simulink library "AeroSim"  (Simulink 7.8)
settings: Solver=ode45  StartTime=0.0  StopTime=10.0  RelTol=1e-3
libraries: AeroSim x13
settings Model: Creator=Ryan  LastModifiedBy=Ryan

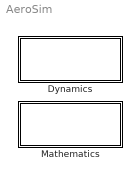
== system AeroSim ==
  Dynamics : Subsystem
      mask Display: disp('Dynamics')
  Mathematics : Subsystem
      mask Display: disp('Mathematics')

== system AeroSim/Dynamics ==
  Equations of Motion : Subsystem
  Rotational EoM : Subsystem
  Translational EoM : Subsystem

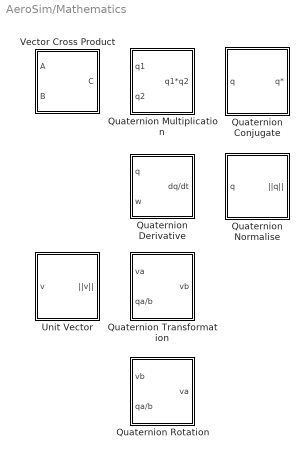
== system AeroSim/Mathematics ==
  Quaternion Conjugate : Subsystem
  Quaternion Derivative : Subsystem
  Quaternion Multiplication : Subsystem
  Quaternion Normalise : Subsystem
  Quaternion Rotation : Subsystem
  Quaternion Transformation : Subsystem
  Unit Vector : Subsystem
  Vector Cross Product : Subsystem

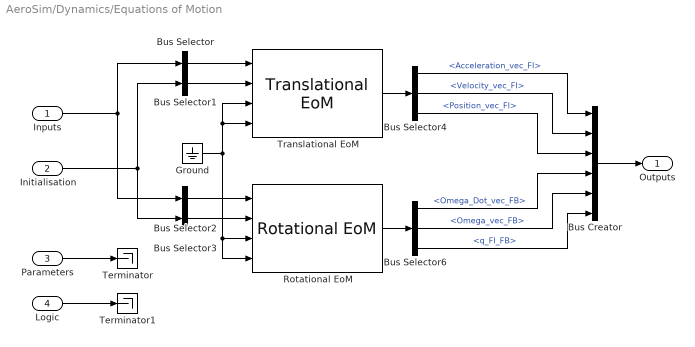
== system AeroSim/Dynamics/Equations of Motion ==
  Inputs : Inport  OutDataTypeStr=Bus: Dynamics_EquationsOfMotion_Inputs
  Initialisation : Inport  Port=2  OutDataTypeStr=Bus: Dynamics_EquationsOfMotion_Initialisation
  Parameters : Inport  Port=3
  Logic : Inport  Port=4
  Bus Creator : BusCreator  Inputs=6
  Bus Selector : BusSelector  OutputSignals=Force_vec_FI,Mass  OutputAsBus=on
  Bus Selector1 : BusSelector  OutputSignals=Ini_Velocity_vec_FI,Ini_Position_vec_FI  OutputAsBus=on
  Bus Selector2 : BusSelector  OutputSignals=Torque_vec_FB,Inertia_mat_FB  OutputAsBus=on
  Bus Selector3 : BusSelector  OutputSignals=Ini_Omega_vec_FB,Ini_q_FI_FB  OutputAsBus=on
  Bus Selector4 : BusSelector  OutputSignals=Acceleration_vec_FI,Velocity_vec_FI,Position_vec_FI
  Bus Selector6 : BusSelector  OutputSignals=Omega_Dot_vec_FB,Omega_vec_FB,q_FI_FB
  Ground : Ground
  Rotational EoM : AeroSim/Dynamics/Rotational EoM
  Terminator : Terminator
  Terminator1 : Terminator
  Translational EoM : AeroSim/Dynamics/Translational EoM
  Outputs : Outport  OutDataTypeStr=Bus: Dynamics_EquationsOfMotion_Outputs
  wires:
  Ground/1 -> Rotational EoM/4, Rotational EoM/3, Translational EoM/4, Translational EoM/3
  Bus Selector3/1 -> Rotational EoM/2
  Bus Selector2/1 -> Rotational EoM/1
  Initialisation/1 -> Bus Selector3/1, Bus Selector1/1
  Bus Selector1/1 -> Translational EoM/2
  Bus Selector/1 -> Translational EoM/1
  Inputs/1 -> Bus Selector2/1, Bus Selector/1
  Bus Creator/1 -> Outputs/1
  Bus Selector4/3 -> Bus Creator/3  "<Position_vec_FI>"
  Bus Selector4/2 -> Bus Creator/2  "<Velocity_vec_FI>"
  Bus Selector4/1 -> Bus Creator/1  "<Acceleration_vec_FI>"
  Bus Selector6/3 -> Bus Creator/6  "<q_FI_FB>"
  Bus Selector6/2 -> Bus Creator/5  "<Omega_vec_FB>"
  Bus Selector6/1 -> Bus Creator/4  "<Omega_Dot_vec_FB>"
  Rotational EoM/1 -> Bus Selector6/1
  Translational EoM/1 -> Bus Selector4/1
  Logic/1 -> Terminator1/1
  Parameters/1 -> Terminator/1

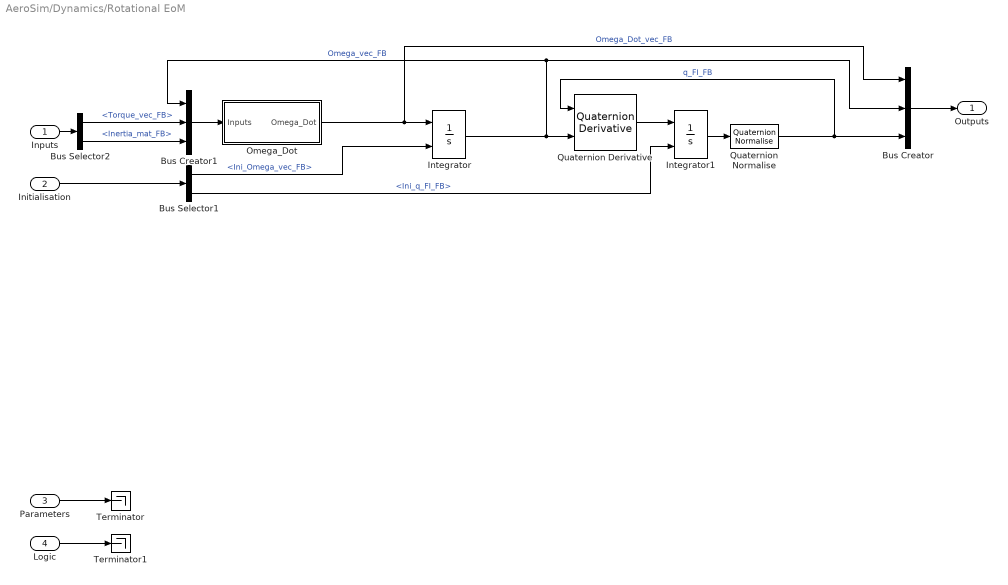
== system AeroSim/Dynamics/Rotational EoM ==
  Inputs : Inport  OutDataTypeStr=Bus: Dynamics_RotationalEoM_Inputs
  Initialisation : Inport  Port=2  OutDataTypeStr=Bus: Dynamics_RotationalEoM_Initialisation
  Parameters : Inport  Port=3
  Logic : Inport  Port=4
  Bus Creator : BusCreator  Inputs=3
  Bus Creator1 : BusCreator  Inputs=3
  Bus Selector1 : BusSelector  OutputSignals=Ini_Omega_vec_FB,Ini_q_FI_FB
  Bus Selector2 : BusSelector  OutputSignals=Torque_vec_FB,Inertia_mat_FB
  Integrator : Integrator  InitialConditionSource=external
  Integrator1 : Integrator  InitialConditionSource=external
  Omega_Dot : Subsystem
  Quaternion Derivative : AeroSim/Mathematics/Quaternion Derivative
  Quaternion Normalise : AeroSim/Mathematics/Quaternion Normalise
  Terminator : Terminator
  Terminator1 : Terminator
  Outputs : Outport  OutDataTypeStr=Bus: Dynamics_RotationalEoM_Outputs
  wires:
  Bus Creator1/1 -> Omega_Dot/1(Inputs)
  Bus Selector2/1 -> Bus Creator1/2  "<Torque_vec_FB>"
  Bus Selector2/2 -> Bus Creator1/3  "<Inertia_mat_FB>"
  Inputs/1 -> Bus Selector2/1
  Quaternion Normalise/1 -> Bus Creator/3, Quaternion Derivative/1  "q_FI_FB"
  Integrator1/1 -> Quaternion Normalise/1
  Bus Selector1/2 -> Integrator1/2  "<Ini_q_FI_FB>"
  Quaternion Derivative/1 -> Integrator1/1
  Integrator/1 -> Bus Creator1/1, Bus Creator/2, Quaternion Derivative/2  "Omega_vec_FB"
  Bus Selector1/1 -> Integrator/2  "<Ini_Omega_vec_FB>"
  Omega_Dot/1(Omega_Dot) -> Bus Creator/1, Integrator/1  "Omega_Dot_vec_FB"
  Bus Creator/1 -> Outputs/1
  Initialisation/1 -> Bus Selector1/1
  Logic/1 -> Terminator1/1
  Parameters/1 -> Terminator/1

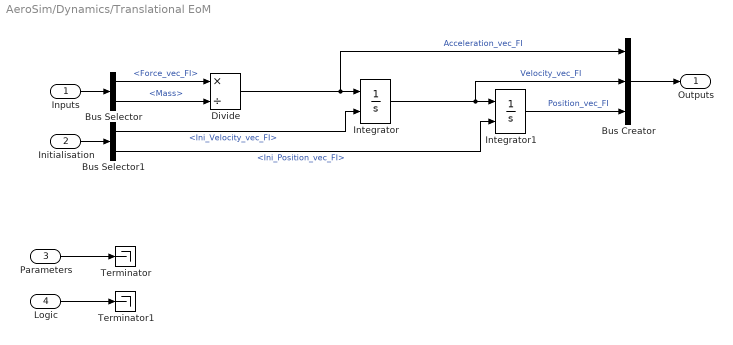
== system AeroSim/Dynamics/Translational EoM ==
  Inputs : Inport  OutDataTypeStr=Bus: Dynamics_TranslationalEoM_Inputs
  Initialisation : Inport  Port=2  OutDataTypeStr=Bus: Dynamics_TranslationalEoM_Initialisation
  Parameters : Inport  Port=3
  Logic : Inport  Port=4
  Bus Creator : BusCreator  Inputs=3
  Bus Selector : BusSelector  OutputSignals=Force_vec_FI,Mass
  Bus Selector1 : BusSelector  OutputSignals=Ini_Velocity_vec_FI,Ini_Position_vec_FI
  Divide : Product  Inputs=*/
  Integrator : Integrator  InitialConditionSource=external
  Integrator1 : Integrator  InitialConditionSource=external
  Terminator : Terminator
  Terminator1 : Terminator
  Outputs : Outport  OutDataTypeStr=Bus: Dynamics_TranslationalEoM_Outputs
  wires:
  Parameters/1 -> Terminator/1
  Logic/1 -> Terminator1/1
  Inputs/1 -> Bus Selector/1
  Bus Selector/1 -> Divide/1  "<Force_vec_FI>"
  Bus Selector/2 -> Divide/2  "<Mass>"
  Initialisation/1 -> Bus Selector1/1
  Bus Creator/1 -> Outputs/1
  Divide/1 -> Integrator/1, Bus Creator/1  "Acceleration_vec_FI"
  Bus Selector1/1 -> Integrator/2  "<Ini_Velocity_vec_FI>"
  Integrator/1 -> Integrator1/1, Bus Creator/2  "Velocity_vec_FI"
  Bus Selector1/2 -> Integrator1/2  "<Ini_Position_vec_FI>"
  Integrator1/1 -> Bus Creator/3  "Position_vec_FI"

== system AeroSim/Mathematics/Quaternion Conjugate ==
  q : Inport
  Demux : Demux  Outputs=[1 3]
  Gain : Gain  Gain=-1
  Mux : Mux  Inputs=2
  q* : Outport
  wires:
  q/1 -> Demux/1
  Demux/2 -> Gain/1
  Demux/1 -> Mux/1
  Gain/1 -> Mux/2
  Mux/1 -> q*/1

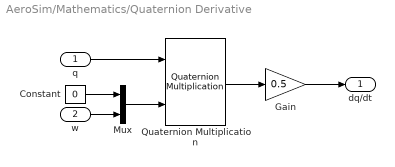
== system AeroSim/Mathematics/Quaternion Derivative ==
  q : Inport
  w : Inport  Port=2
  Constant : Constant  Value=0
  Gain : Gain  Gain=0.5
  Mux : Mux  Inputs=2
  Quaternion Multiplication : AeroSim/Mathematics/Quaternion Multiplication
  dq/dt : Outport
  wires:
  w/1 -> Mux/2
  Constant/1 -> Mux/1
  q/1 -> Quaternion Multiplication/1
  Mux/1 -> Quaternion Multiplication/2
  Quaternion Multiplication/1 -> Gain/1
  Gain/1 -> dq/dt/1

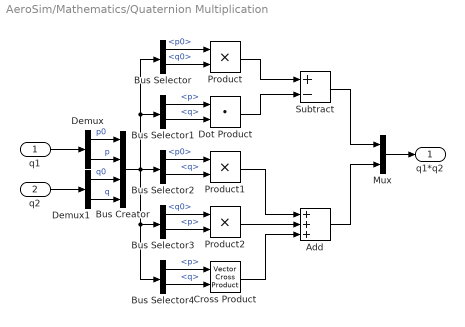
== system AeroSim/Mathematics/Quaternion Multiplication ==
  q1 : Inport
  q2 : Inport  Port=2
  Add : Sum  Inputs=+++
  Bus Creator : BusCreator
  Bus Selector : BusSelector  OutputSignals=p0,q0
  Bus Selector1 : BusSelector  OutputSignals=p,q
  Bus Selector2 : BusSelector  OutputSignals=p0,q
  Bus Selector3 : BusSelector  OutputSignals=q0,p
  Bus Selector4 : BusSelector  OutputSignals=p,q
  Cross Product : AeroSim/Mathematics/Vector Cross Product
  Demux : Demux  Outputs=[1 3]
  Demux1 : Demux  Outputs=[1 3]
  Dot Product : DotProduct  InputSameDT=on  OutDataTypeStr=Inherit: Inherit via internal rule
  Mux : Mux  Inputs=2
  Product : Product  RndMeth=Zero
  Product1 : Product  RndMeth=Zero
  Product2 : Product  RndMeth=Zero
  Subtract : Sum  Inputs=+-
  q1*q2 : Outport
  wires:
  q1/1 -> Demux/1
  q2/1 -> Demux1/1
  Product/1 -> Subtract/1
  Dot Product/1 -> Subtract/2
  Product2/1 -> Add/2
  Product1/1 -> Add/1
  Cross Product/1 -> Add/3
  Subtract/1 -> Mux/1
  Add/1 -> Mux/2
  Mux/1 -> q1*q2/1
  Demux/1 -> Bus Creator/1  "p0"
  Demux/2 -> Bus Creator/2  "p"
  Demux1/1 -> Bus Creator/3  "q0"
  Demux1/2 -> Bus Creator/4  "q"
  Bus Selector/1 -> Product/1  "<p0>"
  Bus Selector/2 -> Product/2  "<q0>"
  Bus Creator/1 -> Bus Selector2/1, Bus Selector/1, Bus Selector1/1, Bus Selector3/1, Bus Selector4/1
  Bus Selector1/1 -> Dot Product/1  "<p>"
  Bus Selector1/2 -> Dot Product/2  "<q>"
  Bus Selector2/1 -> Product1/1  "<p0>"
  Bus Selector2/2 -> Product1/2  "<q>"
  Bus Selector3/1 -> Product2/1  "<q0>"
  Bus Selector3/2 -> Product2/2  "<p>"
  Bus Selector4/1 -> Cross Product/1  "<p>"
  Bus Selector4/2 -> Cross Product/2  "<q>"

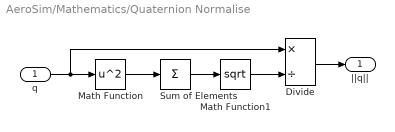
== system AeroSim/Mathematics/Quaternion Normalise ==
  q : Inport
  Divide : Product  Inputs=*/
  Math Function : Math  Operator=square  SaturateOnIntegerOverflow=on
  Math Function1 : Math  Operator=sqrt  SaturateOnIntegerOverflow=on
  Sum of Elements : Sum  Inputs=+
  ||q|| : Outport
  wires:
  q/1 -> Divide/1, Math Function/1
  Divide/1 -> ||q||/1
  Math Function1/1 -> Divide/2
  Sum of Elements/1 -> Math Function1/1
  Math Function/1 -> Sum of Elements/1

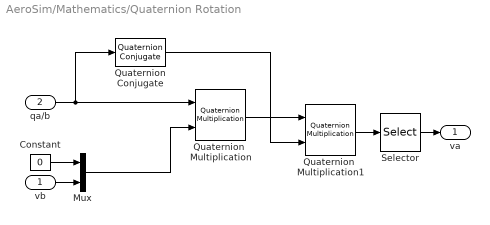
== system AeroSim/Mathematics/Quaternion Rotation ==
  vb : Inport
  qa/b : Inport  Port=2
  Constant : Constant  Value=0
  Mux : Mux  Inputs=2
  Quaternion Conjugate : AeroSim/Mathematics/Quaternion Conjugate
  Quaternion  Multiplication : AeroSim/Mathematics/Quaternion Multiplication
  Quaternion  Multiplication1 : AeroSim/Mathematics/Quaternion Multiplication
  Selector : Selector  InputPortWidth=4  IndexOptions=Index vector (dialog)  Indices=[2 3 4]  OutputSizes=1
  va : Outport
  wires:
  vb/1 -> Mux/2
  Constant/1 -> Mux/1
  qa/b/1 -> Quaternion  Multiplication/1, Quaternion Conjugate/1
  Mux/1 -> Quaternion  Multiplication/2
  Quaternion  Multiplication/1 -> Quaternion  Multiplication1/1
  Quaternion  Multiplication1/1 -> Selector/1
  Selector/1 -> va/1
  Quaternion Conjugate/1 -> Quaternion  Multiplication1/2

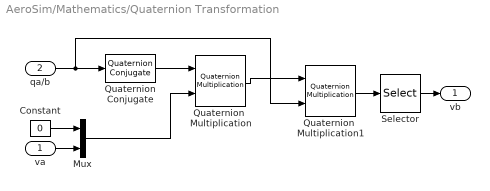
== system AeroSim/Mathematics/Quaternion Transformation ==
  va : Inport
  qa/b : Inport  Port=2
  Constant : Constant  Value=0
  Mux : Mux  Inputs=2
  Quaternion Conjugate : AeroSim/Mathematics/Quaternion Conjugate
  Quaternion  Multiplication : AeroSim/Mathematics/Quaternion Multiplication
  Quaternion  Multiplication1 : AeroSim/Mathematics/Quaternion Multiplication
  Selector : Selector  InputPortWidth=4  IndexOptions=Index vector (dialog)  Indices=[2 3 4]  OutputSizes=1
  vb : Outport
  wires:
  va/1 -> Mux/2
  Constant/1 -> Mux/1
  qa/b/1 -> Quaternion Conjugate/1, Quaternion  Multiplication1/2
  Mux/1 -> Quaternion  Multiplication/2
  Quaternion Conjugate/1 -> Quaternion  Multiplication/1
  Quaternion  Multiplication/1 -> Quaternion  Multiplication1/1
  Quaternion  Multiplication1/1 -> Selector/1
  Selector/1 -> vb/1

== system AeroSim/Mathematics/Unit Vector ==
  v : Inport
  Divide : Product  Inputs=*/
  Math Function : Math  Operator=square  SaturateOnIntegerOverflow=on
  Math Function1 : Math  Operator=sqrt  SaturateOnIntegerOverflow=on
  Sum of Elements : Sum  Inputs=+
  ||v|| : Outport
  wires:
  v/1 -> Divide/1, Math Function/1
  Divide/1 -> ||v||/1
  Math Function1/1 -> Divide/2
  Sum of Elements/1 -> Math Function1/1
  Math Function/1 -> Sum of Elements/1

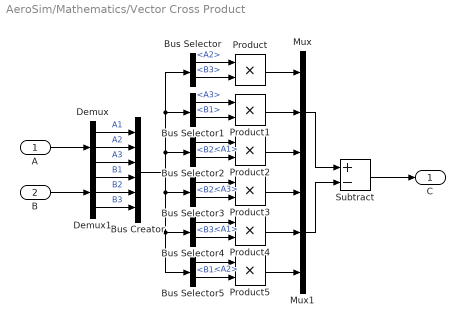
== system AeroSim/Mathematics/Vector Cross Product ==
  A : Inport
  B : Inport  Port=2
  Bus Creator : BusCreator  Inputs=6
  Bus Selector : BusSelector  OutputSignals=A2,B3
  Bus Selector1 : BusSelector  OutputSignals=A3,B1
  Bus Selector2 : BusSelector  OutputSignals=A1,B2
  Bus Selector3 : BusSelector  OutputSignals=A3,B2
  Bus Selector4 : BusSelector  OutputSignals=A1,B3
  Bus Selector5 : BusSelector  OutputSignals=A2,B1
  Demux : Demux  Outputs=3
  Demux1 : Demux  Outputs=3
  Mux : Mux  Inputs=3
  Mux1 : Mux  Inputs=3
  Product{,1..5} (6 alike) : Product  RndMeth=Zero
  Subtract : Sum  Inputs=+-
  C : Outport
  wires:
  Subtract/1 -> C/1
  Bus Creator/1 -> Bus Selector4/1, Bus Selector5/1, Bus Selector3/1, Bus Selector2/1, Bus Selector1/1, Bus Selector/1
  Mux1/1 -> Subtract/2
  Mux/1 -> Subtract/1
  Product5/1 -> Mux1/3
  Product4/1 -> Mux1/2
  Product3/1 -> Mux1/1
  Product2/1 -> Mux/3
  Product1/1 -> Mux/2
  Product/1 -> Mux/1
  Bus Selector5/2 -> Product5/2  "<B1>"
  Bus Selector5/1 -> Product5/1  "<A2>"
  Bus Selector4/2 -> Product4/2  "<B3>"
  Bus Selector4/1 -> Product4/1  "<A1>"
  Bus Selector3/2 -> Product3/2  "<B2>"
  Bus Selector3/1 -> Product3/1  "<A3>"
  Bus Selector2/2 -> Product2/2  "<B2>"
  Bus Selector2/1 -> Product2/1  "<A1>"
  Bus Selector1/2 -> Product1/2  "<B1>"
  Bus Selector1/1 -> Product1/1  "<A3>"
  Bus Selector/2 -> Product/2  "<B3>"
  Bus Selector/1 -> Product/1  "<A2>"
  Demux1/3 -> Bus Creator/6  "B3"
  Demux1/2 -> Bus Creator/5  "B2"
  Demux1/1 -> Bus Creator/4  "B1"
  Demux/3 -> Bus Creator/3  "A3"
  Demux/2 -> Bus Creator/2  "A2"
  Demux/1 -> Bus Creator/1  "A1"
  B/1 -> Demux1/1
  A/1 -> Demux/1

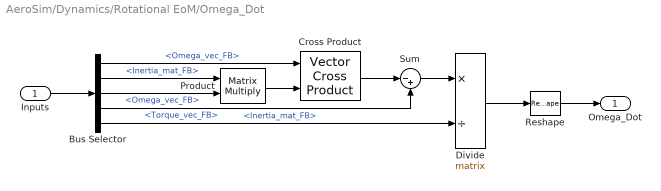
== system AeroSim/Dynamics/Rotational EoM/Omega_Dot ==
  Inputs : Inport
  Bus Selector : BusSelector  OutputSignals=Omega_vec_FB,Inertia_mat_FB,Omega_vec_FB,Torque_vec_FB,Inertia_mat_FB
  Cross Product : AeroSim/Mathematics/Vector Cross Product
  Divide : Product  Inputs=*/  Multiplication=Matrix(*)
  Product : Product  Multiplication=Matrix(*)  RndMeth=Zero
  Reshape : Reshape
  Sum : Sum  Inputs=|-+
  Omega_Dot : Outport
  wires:
  Reshape/1 -> Omega_Dot/1
  Bus Selector/5 -> Divide/2  "<Inertia_mat_FB>"
  Bus Selector/2 -> Product/1  "<Inertia_mat_FB>"
  Divide/1 -> Reshape/1
  Sum/1 -> Divide/1
  Bus Selector/4 -> Sum/2  "<Torque_vec_FB>"
  Bus Selector/3 -> Product/2  "<Omega_vec_FB>"
  Bus Selector/1 -> Cross Product/1  "<Omega_vec_FB>"
  Cross Product/1 -> Sum/1
  Product/1 -> Cross Product/2
  Inputs/1 -> Bus Selector/1
